simulink model "rtwdemo_deadpath"  (Simulink 6.0)
settings: Solver=FixedStepDiscrete  StartTime=0.0  StopTime=10.0  RelTol=1e-3
libraries: rtwdemowidgets x2
settings Model: Creator=The MathWorks Inc.  LastModifiedBy=batserve  ExtModeAutoUpdateStatusClock=off
settings DataIOCC: SaveOutput=off  SaveTime=off  SignalLoggingName=sigsOut
settings OptimizationCC: InlineParams=on  EnforceIntegerDowncast=off  StateBitsets=on  DataBitsets=on  UseTempVars=on
settings DebuggingCC: CheckExecutionContextPreStartOutputMsg=on  CheckExecutionContextRuntimeOutputMsg=on  SolverPrmCheckMsg=none
settings RTWCC: TLCOptions=-p0 -aWarnNonSaturatedBlocks=0  GenerateReport=on  RTWVerbose=off  ProcessScript=grt_make_rtw_hook  LaunchReport=on
settings CodeAppCC: ForceParamTrailComments=on  PrefixModelToSubsysFcnNames=off
settings GRTTargetCC: MatFileLogging=off

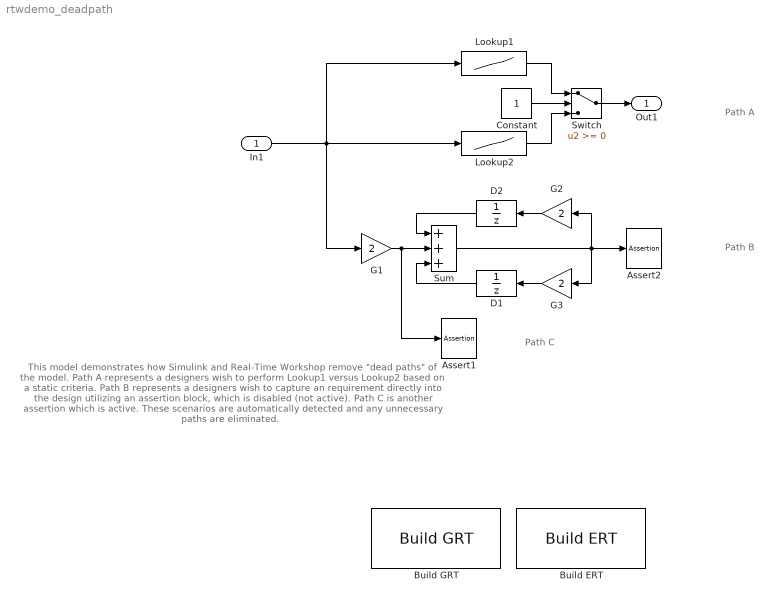
== system rtwdemo_deadpath ==
  note: This model demonstrates how Simulink and Real-Time Workshop remove "dead paths" of the model.
      | Path A represents a designers wish to perform Lookup1 versus Lookup2 based on a static
      | criteria.  Path B represents a designers wish to capture an requirement directly into the
      | design utilizing an assertion block, which is disabled (not active).  Path C is another
      | assertion which is active.  These scenarios are automatically detected and any unnecessary
      | paths are eliminated.
  note: Path A
  note: Path B
  note: Path C
  In1 : Inport  Port=1  LatchInput=off
  Assert1 : Assertion
  Assert2 : Assertion  Enabled=off
  Build ERT : rtwdemowidgets/Build ERT  attrib_overrides={}
  Build GRT : rtwdemowidgets/Build GRT  attrib_overrides={}
  Constant : Constant
  D1 : UnitDelay  Orientation=left
  D2 : UnitDelay  Orientation=left
  G1 : Gain  Gain=2  SaturateOnIntegerOverflow=on
  G2 : Gain  Orientation=left  Gain=2  SaturateOnIntegerOverflow=on
  G3 : Gain  Orientation=left  Gain=2  SaturateOnIntegerOverflow=on
  Lookup1 : Lookup  DialogController=Simulink.DDGSource  InputValues=[-5:5]  OutputValues=tanh([-5:5])  SaturateOnIntegerOverflow=on
  Lookup2 : Lookup  DialogController=Simulink.DDGSource  InputValues=[-5:5]  OutputValues=cosh([-5:5])  SaturateOnIntegerOverflow=on
  Sum : Sum  Inputs=+++  SaturateOnIntegerOverflow=on
  Switch : Switch  SaturateOnIntegerOverflow=on
  Out1 : Outport
  wires:
  Constant/1 -> Switch/2
  Lookup1/1 -> Switch/1
  Lookup2/1 -> Switch/3
  Switch/1 -> Out1/1
  In1/1 -> Lookup1/1, Lookup2/1, G1/1
  G1/1 -> Sum/2, Assert1/1
  D2/1 -> Sum/1
  G2/1 -> D2/1
  D1/1 -> Sum/3
  G3/1 -> D1/1
  Sum/1 -> G3/1, G2/1, Assert2/1
